simulink model "experimentHarnessCurvedLane_CarSim_Interface"  (R2025b)
settings: Solver=FixedStepAuto  StartTime=0.0  StopTime=10  FixedStep=0.0005  MaxStep=tv.maxSolverStep  RelTol=1e-3
undefined symbols (not defined in the file or in its folder): baseline, scenario
libraries: Solver_SF x1
settings Model: Creator=jaiden  LastModifiedBy=r3anjum

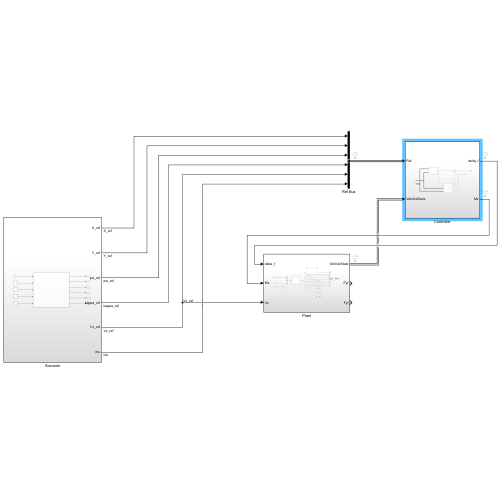
[thumbnail: Simulink's stored preview of the top-level diagram]
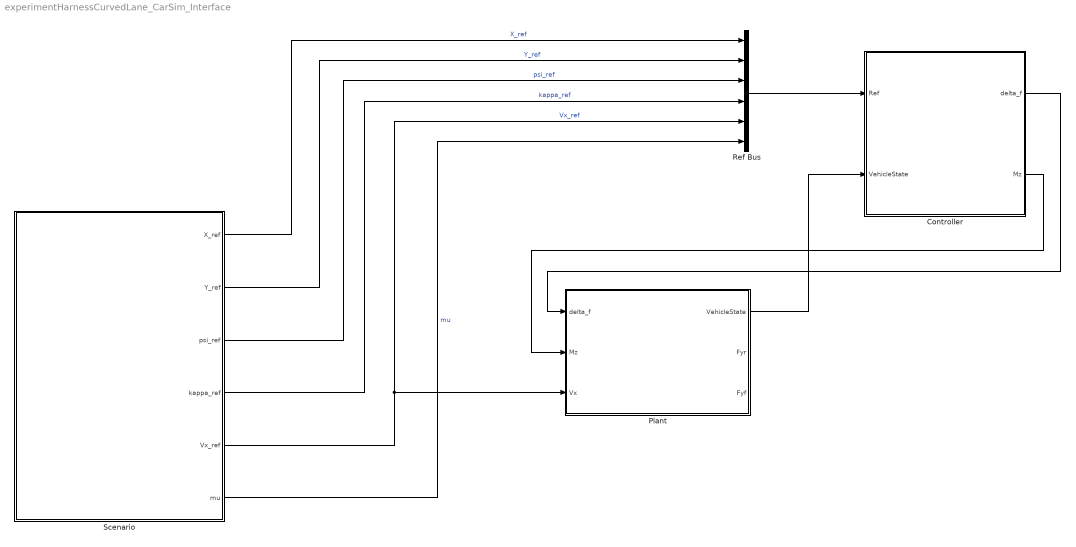
== system experimentHarnessCurvedLane_CarSim_Interface ==
  Controller : Subsystem
  Plant : Subsystem
  Ref Bus : BusCreator  Inputs=6  OutDataTypeStr=Bus: ReferenceBus
  Scenario : Subsystem
  wires:
  Scenario/5(Vx_ref) -> Plant/3(Vx), Ref Bus/5  "Vx_ref"
  Plant/1(VehicleState) -> Controller/2(VehicleState)
  Scenario/1(X_ref) -> Ref Bus/1  "X_ref"
  Scenario/2(Y_ref) -> Ref Bus/2  "Y_ref"
  Scenario/3(psi_ref) -> Ref Bus/3  "psi_ref"
  Scenario/4(kappa_ref) -> Ref Bus/4  "kappa_ref"
  Scenario/6(mu) -> Ref Bus/6  "mu"
  Ref Bus/1 -> Controller/1(Ref)
  Controller/1(delta_f) -> Plant/1(delta_f)
  Controller/2(Mz) -> Plant/2(Mz)

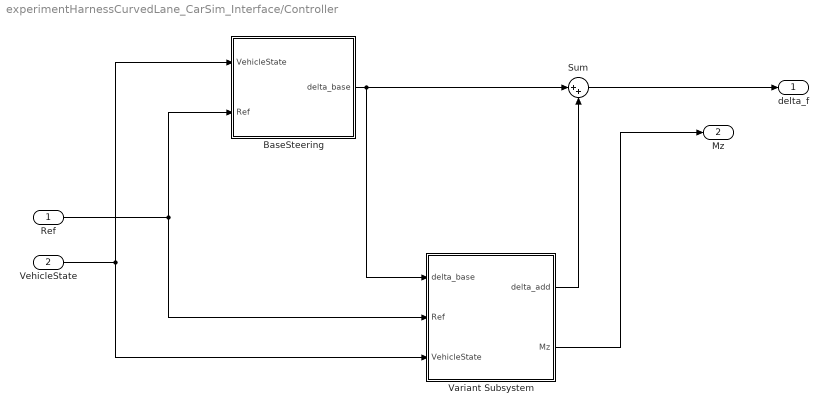
== system experimentHarnessCurvedLane_CarSim_Interface/Controller ==
  Ref : Inport
  VehicleState : Inport  Port=2
  BaseSteering : Subsystem
  Sum : Sum  Inputs=|++
  Variant Subsystem : Subsystem  Variant=on
  delta_f : Outport
  Mz : Outport  Port=2
  wires:
  Ref/1 -> Variant Subsystem/2(Ref), BaseSteering/2(Ref)
  VehicleState/1 -> Variant Subsystem/3(VehicleState), BaseSteering/1(VehicleState)
  BaseSteering/1(delta_base) -> Variant Subsystem/1(delta_base), Sum/1
  Variant Subsystem/1(delta_add) -> Sum/2
  Sum/1 -> delta_f/1
  Variant Subsystem/2(Mz) -> Mz/1

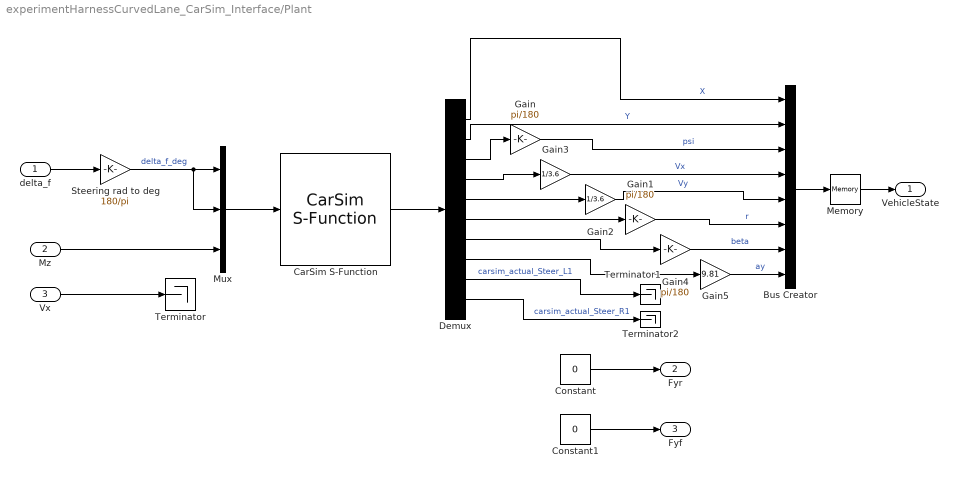
== system experimentHarnessCurvedLane_CarSim_Interface/Plant ==
  delta_f : Inport
  Mz : Inport  Port=2
  Vx : Inport  Port=3
  Bus Creator : BusCreator  Inputs=8  OutDataTypeStr=Bus: VehicleStateBus  NonVirtualBus=on
  CarSim S-Function : Solver_SF/CarSim S-Function  Priority=1  SIMFILE=simfile.sim  Run_RTs=off  vs_state_ind=Run  StopMode_ind=Vehicle Model
  Constant : Constant  Value=0
  Constant1 : Constant  Value=0
  Demux : Demux  Outputs=10
  Gain : Gain  Gain=pi/180
  Gain1 : Gain  Gain=pi/180
  Gain2 : Gain  Gain=1/3.6
  Gain3 : Gain  Gain=1/3.6
  Gain4 : Gain  Gain=pi/180
  Gain5 : Gain  Gain=9.81
  Memory : Memory
  Mux : Mux  Inputs=3
  Steering rad to deg : Gain  Gain=180/pi
  Terminator : Terminator
  Terminator1 : Terminator
  Terminator2 : Terminator
  VehicleState : Outport
  Fyr : Outport  Port=2
  Fyf : Outport  Port=3
  wires:
  delta_f/1 -> Steering rad to deg/1
  Mz/1 -> Mux/3
  Vx/1 -> Terminator/1
  Memory/1 -> VehicleState/1
  Mux/1 -> CarSim S-Function/1
  CarSim S-Function/1 -> Demux/1
  Demux/3 -> Gain/1
  Demux/4 -> Gain3/1
  Demux/5 -> Gain2/1
  Demux/6 -> Gain1/1
  Demux/7 -> Gain4/1
  Demux/8 -> Gain5/1
  Demux/9 -> Terminator1/1  "carsim_actual_Steer_L1"
  Demux/10 -> Terminator2/1  "carsim_actual_Steer_R1"
  Gain5/1 -> Bus Creator/8  "ay"
  Gain4/1 -> Bus Creator/7  "beta"
  Gain1/1 -> Bus Creator/6  "r"
  Gain2/1 -> Bus Creator/5  "Vy"
  Gain3/1 -> Bus Creator/4  "Vx"
  Gain/1 -> Bus Creator/3  "psi"
  Demux/1 -> Bus Creator/1  "X"
  Demux/2 -> Bus Creator/2  "Y"
  Bus Creator/1 -> Memory/1
  Constant/1 -> Fyr/1
  Constant1/1 -> Fyf/1
  Steering rad to deg/1 -> Mux/2, Mux/1  "delta_f_deg"

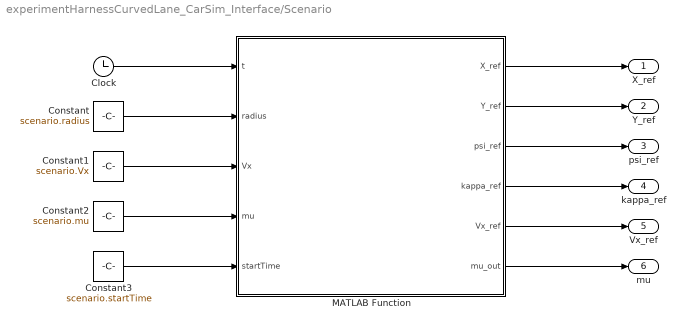
== system experimentHarnessCurvedLane_CarSim_Interface/Scenario ==
  Clock : Clock
  Constant : Constant  Value=scenario.radius
  Constant1 : Constant  Value=scenario.Vx
  Constant2 : Constant  Value=scenario.mu
  Constant3 : Constant  Value=scenario.startTime
  MATLAB Function : MATLAB Function  TreatAsAtomicUnit=on
  X_ref : Outport
  Y_ref : Outport  Port=2
  psi_ref : Outport  Port=3
  kappa_ref : Outport  Port=4
  Vx_ref : Outport  Port=5
  mu : Outport  Port=6
  wires:
  Clock/1 -> MATLAB Function/1(t)
  Constant/1 -> MATLAB Function/2(radius)
  Constant1/1 -> MATLAB Function/3(Vx)
  Constant2/1 -> MATLAB Function/4(mu)
  Constant3/1 -> MATLAB Function/5(startTime)
  MATLAB Function/1(X_ref) -> X_ref/1
  MATLAB Function/2(Y_ref) -> Y_ref/1
  MATLAB Function/3(psi_ref) -> psi_ref/1
  MATLAB Function/4(kappa_ref) -> kappa_ref/1
  MATLAB Function/5(Vx_ref) -> Vx_ref/1
  MATLAB Function/6(mu_out) -> mu/1

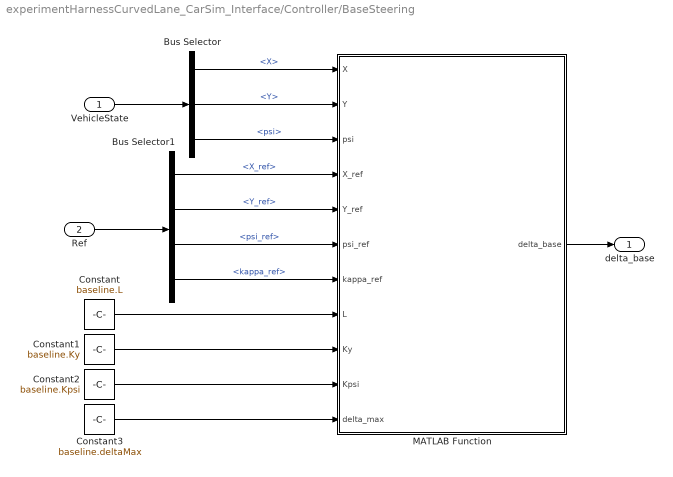
== system experimentHarnessCurvedLane_CarSim_Interface/Controller/BaseSteering ==
  VehicleState : Inport  OutDataTypeStr=Bus: VehicleStateBus
  Ref : Inport  Port=2  OutDataTypeStr=Bus: ReferenceBus
  Bus Selector : BusSelector  OutputSignals=X,Y,psi
  Bus Selector1 : BusSelector  OutputSignals=X_ref,Y_ref,psi_ref,kappa_ref
  Constant : Constant  Value=baseline.L
  Constant1 : Constant  Value=baseline.Ky
  Constant2 : Constant  Value=baseline.Kpsi
  Constant3 : Constant  Value=baseline.deltaMax  VectorParams1D=off
  MATLAB Function : MATLAB Function  TreatAsAtomicUnit=on
  delta_base : Outport
  wires:
  VehicleState/1 -> Bus Selector/1
  Ref/1 -> Bus Selector1/1
  Bus Selector/1 -> MATLAB Function/1(X)  "<X>"
  Bus Selector/2 -> MATLAB Function/2(Y)  "<Y>"
  Bus Selector/3 -> MATLAB Function/3(psi)  "<psi>"
  Bus Selector1/1 -> MATLAB Function/4(X_ref)  "<X_ref>"
  Bus Selector1/2 -> MATLAB Function/5(Y_ref)  "<Y_ref>"
  Bus Selector1/3 -> MATLAB Function/6(psi_ref)  "<psi_ref>"
  Bus Selector1/4 -> MATLAB Function/7(kappa_ref)  "<kappa_ref>"
  Constant/1 -> MATLAB Function/8(L)
  Constant1/1 -> MATLAB Function/9(Ky)
  Constant2/1 -> MATLAB Function/10(Kpsi)
  Constant3/1 -> MATLAB Function/11(delta_max)
  MATLAB Function/1(delta_base) -> delta_base/1

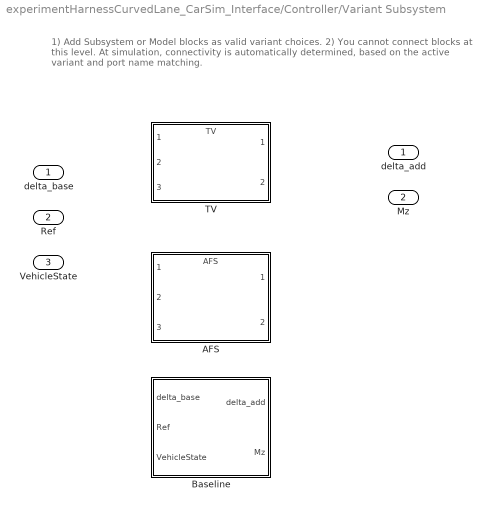
== system experimentHarnessCurvedLane_CarSim_Interface/Controller/Variant Subsystem ==
  note: 1) Add Subsystem or Model blocks as valid variant choices.
      | 2) You cannot connect blocks at this level. At simulation, connectivity is automatically
      | determined, based on the active variant and port name matching.
  delta_base : Inport
  Ref : Inport  Port=2
  VehicleState : Inport  Port=3
  AFS : ModelReference  ModelNameDialog=AFS.slx  SimulationMode=Normal  VariantControl=Choice_1  ModelReferenceVersion=1.11
  Baseline : Subsystem  VariantControl=Choice_2
  TV : ModelReference  ModelNameDialog=TV.slx  SimulationMode=Normal  VariantControl=Choice  ModelReferenceVersion=1.14
  delta_add : Outport
  Mz : Outport  Port=2

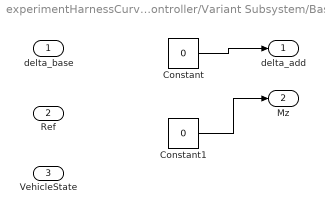
== system experimentHarnessCurvedLane_CarSim_Interface/Controller/Variant Subsystem/Baseline ==
  delta_base : Inport
  Ref : Inport  Port=2  OutDataTypeStr=Bus: ReferenceBus
  VehicleState : Inport  Port=3  OutDataTypeStr=Bus: VehicleStateBus
  Constant : Constant  Value=0
  Constant1 : Constant  Value=0
  delta_add : Outport
  Mz : Outport  Port=2
  wires:
  Constant/1 -> delta_add/1
  Constant1/1 -> Mz/1

== matlab function experimentHarnessCurvedLane_CarSim_Interface/Controller/BaseSteering/MATLAB Function ==
  data: X input; delta_base output; Y input; psi input; X_ref input; Y_ref input; psi_ref input; kappa_ref input; L input; Ky input; Kpsi input; delta_max input
function delta_base = baseSteering( ...
    X, Y, psi, X_ref, Y_ref, psi_ref, kappa_ref, ...
    L, Ky, Kpsi, delta_max)

% Feedforward steering required by the path curvature
delta_ff = atan(L*kappa_ref);

% Signed lateral position error
e_y = -sin(psi_ref)*(X - X_ref) ...
      + cos(psi_ref)*(Y - Y_ref);

% Wrapped heading error in [-pi, pi]
e_psi = atan2(sin(psi_ref - psi), ...
              cos(psi_ref - psi));

% Feedforward plus feedback steering
delta_cmd = delta_ff - Ky*e_y + Kpsi*e_psi;

% Steering-angle limit
delta_base = min(max(delta_cmd, -delta_max), delta_max);

end

== matlab function experimentHarnessCurvedLane_CarSim_Interface/Scenario/MATLAB Function ==
  data: t input; X_ref output; radius input; Vx input; mu input; startTime input; Y_ref output; psi_ref output; kappa_ref output; Vx_ref output; mu_out output
function [X_ref, Y_ref, psi_ref, kappa_ref, Vx_ref, mu_out] = ...
    curvedLaneReference(t, radius, Vx, mu, startTime)

Vx_ref = Vx;
mu_out = mu;

if t < startTime
    % Initial straight section
    X_ref = Vx*t;
    Y_ref = 0;
    psi_ref = 0;
    kappa_ref = 0;
else
    % Constant-radius curved section
    X0 = Vx*startTime;
    theta = Vx*(t - startTime)/radius;

    X_ref = X0 + radius*sin(theta);
    Y_ref = radius*(1 - cos(theta));
    psi_ref = theta;
    kappa_ref = 1/radius;
end

end
